simulink model "ban1"  (R2018b)
settings: Solver=FixedStepAuto  StartTime=0.0  StopTime=100  FixedStep=0.001  RelTol=1e-3
settings Model: Creator=User  LastModifiedBy=User

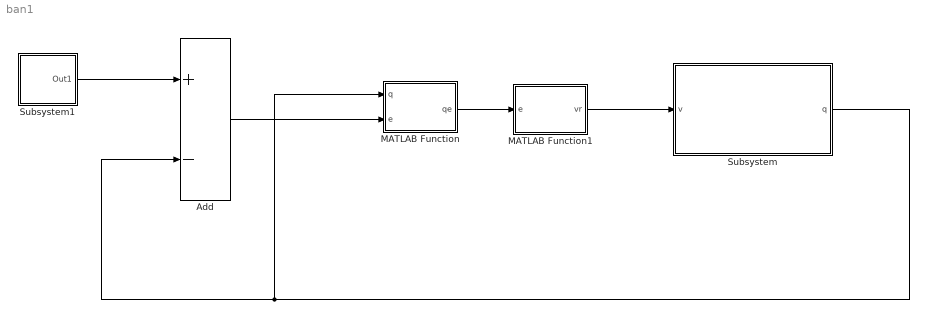
== system ban1 ==
  Add : Sum  Inputs=+-
  MATLAB Function : MATLAB Function  TreatAsAtomicUnit=on
  MATLAB Function1 : MATLAB Function  TreatAsAtomicUnit=on
  Subsystem : Subsystem
  Subsystem1 : Subsystem
  wires:
  Subsystem1/1(Out1) -> Add/1
  Subsystem/1(q) -> MATLAB Function/1(q), Add/2
  Add/1 -> MATLAB Function/2(e)
  MATLAB Function/1(qe) -> MATLAB Function1/1(e)
  MATLAB Function1/1(vr) -> Subsystem/1(v)

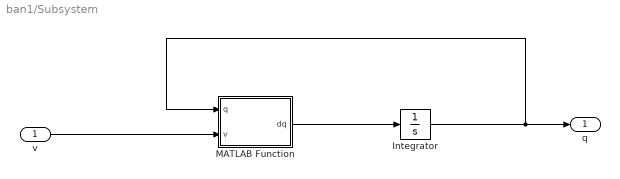
== system ban1/Subsystem ==
  v : Inport
  Integrator : Integrator  InitialCondition=[1.8852;-0.2772;1.1781]
  MATLAB Function : MATLAB Function  TreatAsAtomicUnit=on
  q : Outport
  wires:
  Integrator/1 -> MATLAB Function/1(q), q/1
  MATLAB Function/1(dq) -> Integrator/1
  v/1 -> MATLAB Function/2(v)

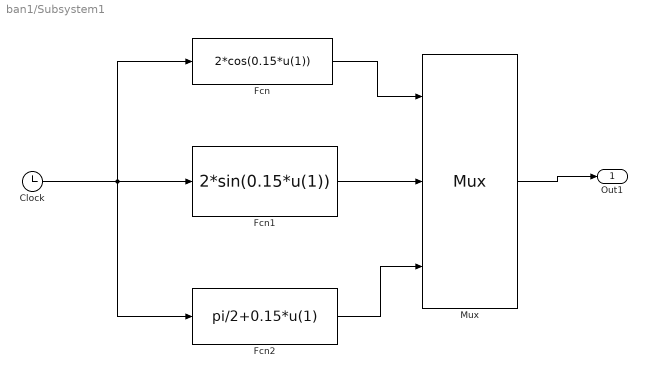
== system ban1/Subsystem1 ==
  Clock : Clock
  Fcn : Fcn  Expr=2*cos(0.15*u(1))
  Fcn1 : Fcn  Expr=2*sin(0.15*u(1))
  Fcn2 : Fcn  Expr=pi/2+0.15*u(1)
  Mux : Mux  Inputs=3
  Out1 : Outport
  wires:
  Clock/1 -> Fcn2/1, Fcn1/1, Fcn/1
  Fcn/1 -> Mux/1
  Fcn1/1 -> Mux/2
  Fcn2/1 -> Mux/3
  Mux/1 -> Out1/1

== matlab function ban1/MATLAB Function ==
  data: q input; qe output; e input
function qe = fcn(q,e)
phi=q(3);
qe=[cos(phi) sin(phi) 0;-sin(phi) cos(phi) 0;0 0 1]*e;
end

== matlab function ban1/Subsystem/MATLAB Function ==
  data: q input; dq output; v input
function dq = fcn(q,v)
phi=q(3);
S=[cos(phi) 0;sin(phi) 0;0 1];
dq=S*v;
end

== matlab function ban1/MATLAB Function1 ==
  data: e input; vr output
function vr=fcn(e)
vr=[0.3*cos(e(3))+10*e(1);
    0.15+10*0.3*e(2)+10*0.3*sin(e(3))];
end
